simulink model "TrackShift_F1_HEV"  (R2025a)
settings: Solver=FixedStepDiscrete  StartTime=0.0  StopTime=90  FixedStep=0.25  RelTol=1e-3
model workspace (MAT data in the model file):
  TS_BRAKE = [0 0.25 0.5 0.75 1 1.25 1.5 1.75 2 2.25 2.5 2.75 ... (722 elements, 361x2)]
  TS_ENGINE_CAPACITY_L = 1.6
  TS_GAP_S = [0 0.25 0.5 0.75 1 1.25 1.5 1.75 2 2.25 2.5 2.75 ... (722 elements, 361x2)]
  TS_GRADIENT_RAD = [0 0.25 0.5 0.75 1 1.25 1.5 1.75 2 2.25 2.5 2.75 ... (722 elements, 361x2)]
  TS_HANDOVER_SOURCE = 'handover.rar / handover/export/models (production logistic models)'
  TS_SAMPLE_TIME_S = 0.25
  TS_SPEED_KPH = [0 0.25 0.5 0.75 1 1.25 1.5 1.75 2 2.25 2.5 2.75 ... (722 elements, 361x2)]
  TS_THROTTLE = [0 0.25 0.5 0.75 1 1.25 1.5 1.75 2 2.25 2.5 2.75 ... (722 elements, 361x2)]
  TS_TRACK_POS_M = [0 0.25 0.5 0.75 1 1.25 1.5 1.75 2 2.25 2.5 2.75 ... (722 elements, 361x2)]
(part 2 of 2)

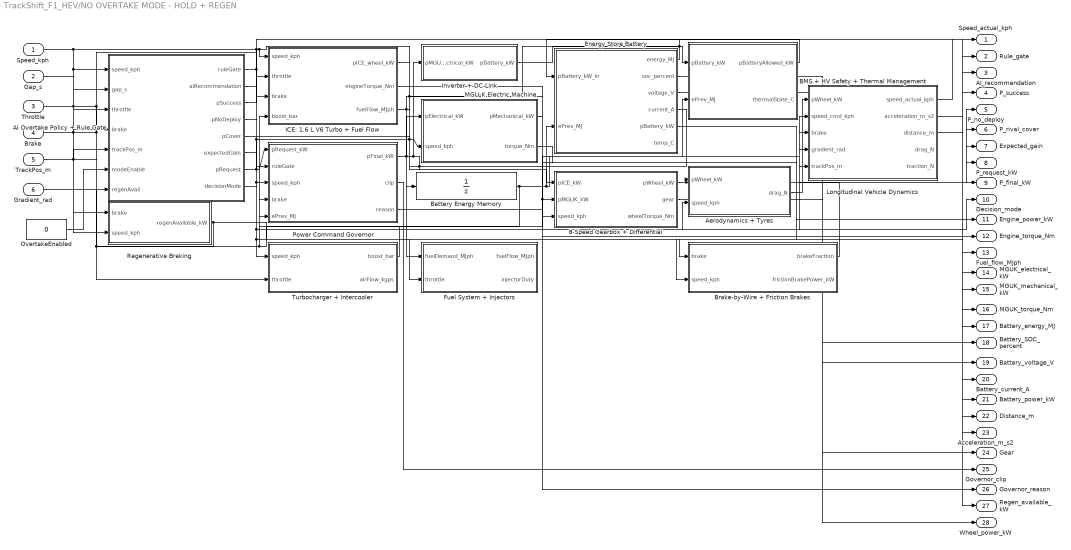
== system TrackShift_F1_HEV/NO OVERTAKE MODE - HOLD + REGEN ==
  Speed_kph : Inport
  Gap_s : Inport  Port=2
  Throttle : Inport  Port=3
  Brake : Inport  Port=4
  TrackPos_m : Inport  Port=5
  Gradient_rad : Inport  Port=6
  8-Speed Gearbox + Differential : MATLAB Function  TreatAsAtomicUnit=on
  AI Overtake Policy + Rule Gate : MATLAB Function  TreatAsAtomicUnit=on
  Aerodynamics + Tyres : MATLAB Function  TreatAsAtomicUnit=on
  BMS + HV Safety + Thermal Management : MATLAB Function  TreatAsAtomicUnit=on
  Battery Energy Memory : UnitDelay  InitialCondition=11.52  SampleTime=0.25  HasFrameUpgradeWarning=on
  Brake-by-Wire + Friction Brakes : MATLAB Function  TreatAsAtomicUnit=on
  Energy Store Battery : MATLAB Function  TreatAsAtomicUnit=on
  Fuel System + Injectors : MATLAB Function  TreatAsAtomicUnit=on
  ICE: 1.6 L V6 Turbo + Fuel Flow : MATLAB Function  TreatAsAtomicUnit=on
  Inverter + DC Link : MATLAB Function  TreatAsAtomicUnit=on
  Longitudinal Vehicle Dynamics : MATLAB Function  TreatAsAtomicUnit=on
  MGU-K Electric Machine : MATLAB Function  TreatAsAtomicUnit=on
  OvertakeEnabled : Constant  Value=0
  Power Command Governor : MATLAB Function  TreatAsAtomicUnit=on
  Regenerative Braking : MATLAB Function  TreatAsAtomicUnit=on
  Turbocharger + Intercooler : MATLAB Function  TreatAsAtomicUnit=on
  Speed_actual_kph : Outport
  Rule_gate : Outport  Port=2
  AI_recommendation : Outport  Port=3
  P_success : Outport  Port=4
  P_no_deploy : Outport  Port=5
  P_rival_cover : Outport  Port=6
  Expected_gain : Outport  Port=7
  P_request_kW : Outport  Port=8
  P_final_kW : Outport  Port=9
  Decision_mode : Outport  Port=10
  Engine_power_kW : Outport  Port=11
  Engine_torque_Nm : Outport  Port=12
  Fuel_flow_MJph : Outport  Port=13
  MGUK_electrical_kW : Outport  Port=14
  MGUK_mechanical_kW : Outport  Port=15
  MGUK_torque_Nm : Outport  Port=16
  Battery_energy_MJ : Outport  Port=17
  Battery_SOC_percent : Outport  Port=18
  Battery_voltage_V : Outport  Port=19
  Battery_current_A : Outport  Port=20
  Battery_power_kW : Outport  Port=21
  Distance_m : Outport  Port=22
  Acceleration_m_s2 : Outport  Port=23
  Gear : Outport  Port=24
  Governor_clip : Outport  Port=25
  Governor_reason : Outport  Port=26
  Regen_available_kW : Outport  Port=27
  Wheel_power_kW : Outport  Port=28
  wires:
  ? -> ?
  Speed_kph/1 -> AI Overtake Policy + Rule Gate/1(speed_kph), Regenerative Braking/2(speed_kph), Turbocharger + Intercooler/1(speed_kph), Brake-by-Wire + Friction Brakes/2(speed_kph), Aerodynamics + Tyres/2(speed_kph), Power Command Governor/3(speed_kph), MGU-K Electric Machine/2(speed_kph), 8-Speed Gearbox + Differential/3(speed_kph), ICE: 1.6 L V6 Turbo + Fuel Flow/1(speed_kph), Longitudinal Vehicle Dynamics/2(speed_cmd_kph)
  Gap_s/1 -> AI Overtake Policy + Rule Gate/2(gap_s)
  Throttle/1 -> Turbocharger + Intercooler/2(throttle), Fuel System + Injectors/2(throttle), ICE: 1.6 L V6 Turbo + Fuel Flow/2(throttle), AI Overtake Policy + Rule Gate/3(throttle)
  Brake/1 -> Power Command Governor/4(brake), Brake-by-Wire + Friction Brakes/1(brake), ICE: 1.6 L V6 Turbo + Fuel Flow/3(brake), AI Overtake Policy + Rule Gate/4(brake), Regenerative Braking/1(brake)
  TrackPos_m/1 -> AI Overtake Policy + Rule Gate/5(trackPos_m), Longitudinal Vehicle Dynamics/5(trackPos_m)
  OvertakeEnabled/1 -> AI Overtake Policy + Rule Gate/6(modeEnable)
  Regenerative Braking/1(regenAvailable_kW) -> AI Overtake Policy + Rule Gate/7(regenAvail), Regen_available_kW/1
  Turbocharger + Intercooler/1(boost_bar) -> ICE: 1.6 L V6 Turbo + Fuel Flow/4(boost_bar)
  ICE: 1.6 L V6 Turbo + Fuel Flow/3(fuelFlow_MJph) -> Fuel System + Injectors/1(fuelDemand_MJph), Fuel_flow_MJph/1
  AI Overtake Policy + Rule Gate/7(pRequest) -> Power Command Governor/1(pRequest_kW), P_request_kW/1
  AI Overtake Policy + Rule Gate/1(ruleGate) -> Power Command Governor/2(ruleGate), Rule_gate/1
  Battery Energy Memory/1 -> Energy Store Battery/2(ePrev_MJ), BMS + HV Safety + Thermal Management/2(ePrev_MJ), Power Command Governor/5(ePrev_MJ)
  Power Command Governor/1(pFinal_kW) -> P_final_kW/1, MGUK_electrical_kW/1, Inverter + DC Link/1(pMGUK_electrical_kW), MGU-K Electric Machine/1(pElectrical_kW)
  Inverter + DC Link/1(pBattery_kW) -> BMS + HV Safety + Thermal Management/1(pBattery_kW)
  BMS + HV Safety + Thermal Management/1(pBatteryAllowed_kW) -> Energy Store Battery/1(pBattery_kW_in)
  Energy Store Battery/1(energy_MJ) -> Battery Energy Memory/1, Battery_energy_MJ/1
  ICE: 1.6 L V6 Turbo + Fuel Flow/1(pICE_wheel_kW) -> 8-Speed Gearbox + Differential/1(pICE_kW), Engine_power_kW/1
  MGU-K Electric Machine/1(pMechanical_kW) -> 8-Speed Gearbox + Differential/2(pMGUK_kW), MGUK_mechanical_kW/1
  8-Speed Gearbox + Differential/1(pWheel_kW) -> Aerodynamics + Tyres/1(pWheel_kW), Wheel_power_kW/1
  Aerodynamics + Tyres/1(drag_N) -> Longitudinal Vehicle Dynamics/1(pWheel_kW)
  Brake-by-Wire + Friction Brakes/1(brakeFraction) -> Longitudinal Vehicle Dynamics/3(brake)
  Gradient_rad/1 -> Longitudinal Vehicle Dynamics/4(gradient_rad)
  Longitudinal Vehicle Dynamics/1(speed_actual_kph) -> Speed_actual_kph/1
  AI Overtake Policy + Rule Gate/2(aiRecommendation) -> AI_recommendation/1
  AI Overtake Policy + Rule Gate/3(pSuccess) -> P_success/1
  AI Overtake Policy + Rule Gate/4(pNoDeploy) -> P_no_deploy/1
  AI Overtake Policy + Rule Gate/5(pCover) -> P_rival_cover/1
  AI Overtake Policy + Rule Gate/6(expectedGain) -> Expected_gain/1
  AI Overtake Policy + Rule Gate/8(decisionMode) -> Decision_mode/1
  ICE: 1.6 L V6 Turbo + Fuel Flow/2(engineTorque_Nm) -> Engine_torque_Nm/1
  MGU-K Electric Machine/2(torque_Nm) -> MGUK_torque_Nm/1
  Energy Store Battery/2(soc_percent) -> Battery_SOC_percent/1
  Energy Store Battery/3(voltage_V) -> Battery_voltage_V/1
  Energy Store Battery/4(current_A) -> Battery_current_A/1
  Energy Store Battery/5(pBattery_kW) -> Battery_power_kW/1
  Longitudinal Vehicle Dynamics/3(distance_m) -> Distance_m/1
  Longitudinal Vehicle Dynamics/2(acceleration_m_s2) -> Acceleration_m_s2/1
  8-Speed Gearbox + Differential/2(gear) -> Gear/1
  Power Command Governor/2(clip) -> Governor_clip/1
  Power Command Governor/3(reason) -> Governor_reason/1

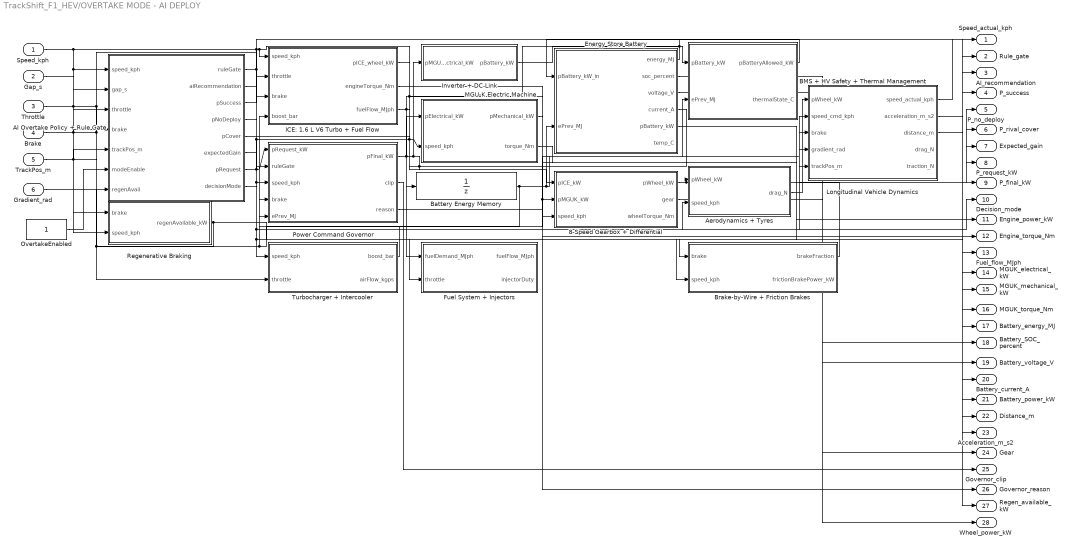
== system TrackShift_F1_HEV/OVERTAKE MODE - AI DEPLOY ==
  Speed_kph : Inport
  Gap_s : Inport  Port=2
  Throttle : Inport  Port=3
  Brake : Inport  Port=4
  TrackPos_m : Inport  Port=5
  Gradient_rad : Inport  Port=6
  8-Speed Gearbox + Differential : MATLAB Function  TreatAsAtomicUnit=on
  AI Overtake Policy + Rule Gate : MATLAB Function  TreatAsAtomicUnit=on
  Aerodynamics + Tyres : MATLAB Function  TreatAsAtomicUnit=on
  BMS + HV Safety + Thermal Management : MATLAB Function  TreatAsAtomicUnit=on
  Battery Energy Memory : UnitDelay  InitialCondition=11.52  SampleTime=0.25  HasFrameUpgradeWarning=on
  Brake-by-Wire + Friction Brakes : MATLAB Function  TreatAsAtomicUnit=on
  Energy Store Battery : MATLAB Function  TreatAsAtomicUnit=on
  Fuel System + Injectors : MATLAB Function  TreatAsAtomicUnit=on
  ICE: 1.6 L V6 Turbo + Fuel Flow : MATLAB Function  TreatAsAtomicUnit=on
  Inverter + DC Link : MATLAB Function  TreatAsAtomicUnit=on
  Longitudinal Vehicle Dynamics : MATLAB Function  TreatAsAtomicUnit=on
  MGU-K Electric Machine : MATLAB Function  TreatAsAtomicUnit=on
  OvertakeEnabled : Constant
  Power Command Governor : MATLAB Function  TreatAsAtomicUnit=on
  Regenerative Braking : MATLAB Function  TreatAsAtomicUnit=on
  Turbocharger + Intercooler : MATLAB Function  TreatAsAtomicUnit=on
  Speed_actual_kph : Outport
  Rule_gate : Outport  Port=2
  AI_recommendation : Outport  Port=3
  P_success : Outport  Port=4
  P_no_deploy : Outport  Port=5
  P_rival_cover : Outport  Port=6
  Expected_gain : Outport  Port=7
  P_request_kW : Outport  Port=8
  P_final_kW : Outport  Port=9
  Decision_mode : Outport  Port=10
  Engine_power_kW : Outport  Port=11
  Engine_torque_Nm : Outport  Port=12
  Fuel_flow_MJph : Outport  Port=13
  MGUK_electrical_kW : Outport  Port=14
  MGUK_mechanical_kW : Outport  Port=15
  MGUK_torque_Nm : Outport  Port=16
  Battery_energy_MJ : Outport  Port=17
  Battery_SOC_percent : Outport  Port=18
  Battery_voltage_V : Outport  Port=19
  Battery_current_A : Outport  Port=20
  Battery_power_kW : Outport  Port=21
  Distance_m : Outport  Port=22
  Acceleration_m_s2 : Outport  Port=23
  Gear : Outport  Port=24
  Governor_clip : Outport  Port=25
  Governor_reason : Outport  Port=26
  Regen_available_kW : Outport  Port=27
  Wheel_power_kW : Outport  Port=28
  wires:
  ? -> ?
  Speed_kph/1 -> AI Overtake Policy + Rule Gate/1(speed_kph), Regenerative Braking/2(speed_kph), Turbocharger + Intercooler/1(speed_kph), Brake-by-Wire + Friction Brakes/2(speed_kph), Aerodynamics + Tyres/2(speed_kph), Power Command Governor/3(speed_kph), MGU-K Electric Machine/2(speed_kph), 8-Speed Gearbox + Differential/3(speed_kph), ICE: 1.6 L V6 Turbo + Fuel Flow/1(speed_kph), Longitudinal Vehicle Dynamics/2(speed_cmd_kph)
  Gap_s/1 -> AI Overtake Policy + Rule Gate/2(gap_s)
  Throttle/1 -> Turbocharger + Intercooler/2(throttle), Fuel System + Injectors/2(throttle), ICE: 1.6 L V6 Turbo + Fuel Flow/2(throttle), AI Overtake Policy + Rule Gate/3(throttle)
  Brake/1 -> Power Command Governor/4(brake), Brake-by-Wire + Friction Brakes/1(brake), ICE: 1.6 L V6 Turbo + Fuel Flow/3(brake), AI Overtake Policy + Rule Gate/4(brake), Regenerative Braking/1(brake)
  TrackPos_m/1 -> AI Overtake Policy + Rule Gate/5(trackPos_m), Longitudinal Vehicle Dynamics/5(trackPos_m)
  OvertakeEnabled/1 -> AI Overtake Policy + Rule Gate/6(modeEnable)
  Regenerative Braking/1(regenAvailable_kW) -> AI Overtake Policy + Rule Gate/7(regenAvail), Regen_available_kW/1
  Turbocharger + Intercooler/1(boost_bar) -> ICE: 1.6 L V6 Turbo + Fuel Flow/4(boost_bar)
  ICE: 1.6 L V6 Turbo + Fuel Flow/3(fuelFlow_MJph) -> Fuel System + Injectors/1(fuelDemand_MJph), Fuel_flow_MJph/1
  AI Overtake Policy + Rule Gate/7(pRequest) -> Power Command Governor/1(pRequest_kW), P_request_kW/1
  AI Overtake Policy + Rule Gate/1(ruleGate) -> Power Command Governor/2(ruleGate), Rule_gate/1
  Battery Energy Memory/1 -> Energy Store Battery/2(ePrev_MJ), BMS + HV Safety + Thermal Management/2(ePrev_MJ), Power Command Governor/5(ePrev_MJ)
  Power Command Governor/1(pFinal_kW) -> P_final_kW/1, MGUK_electrical_kW/1, Inverter + DC Link/1(pMGUK_electrical_kW), MGU-K Electric Machine/1(pElectrical_kW)
  Inverter + DC Link/1(pBattery_kW) -> BMS + HV Safety + Thermal Management/1(pBattery_kW)
  BMS + HV Safety + Thermal Management/1(pBatteryAllowed_kW) -> Energy Store Battery/1(pBattery_kW_in)
  Energy Store Battery/1(energy_MJ) -> Battery Energy Memory/1, Battery_energy_MJ/1
  ICE: 1.6 L V6 Turbo + Fuel Flow/1(pICE_wheel_kW) -> 8-Speed Gearbox + Differential/1(pICE_kW), Engine_power_kW/1
  MGU-K Electric Machine/1(pMechanical_kW) -> 8-Speed Gearbox + Differential/2(pMGUK_kW), MGUK_mechanical_kW/1
  8-Speed Gearbox + Differential/1(pWheel_kW) -> Aerodynamics + Tyres/1(pWheel_kW), Wheel_power_kW/1
  Aerodynamics + Tyres/1(drag_N) -> Longitudinal Vehicle Dynamics/1(pWheel_kW)
  Brake-by-Wire + Friction Brakes/1(brakeFraction) -> Longitudinal Vehicle Dynamics/3(brake)
  Gradient_rad/1 -> Longitudinal Vehicle Dynamics/4(gradient_rad)
  Longitudinal Vehicle Dynamics/1(speed_actual_kph) -> Speed_actual_kph/1
  AI Overtake Policy + Rule Gate/2(aiRecommendation) -> AI_recommendation/1
  AI Overtake Policy + Rule Gate/3(pSuccess) -> P_success/1
  AI Overtake Policy + Rule Gate/4(pNoDeploy) -> P_no_deploy/1
  AI Overtake Policy + Rule Gate/5(pCover) -> P_rival_cover/1
  AI Overtake Policy + Rule Gate/6(expectedGain) -> Expected_gain/1
  AI Overtake Policy + Rule Gate/8(decisionMode) -> Decision_mode/1
  ICE: 1.6 L V6 Turbo + Fuel Flow/2(engineTorque_Nm) -> Engine_torque_Nm/1
  MGU-K Electric Machine/2(torque_Nm) -> MGUK_torque_Nm/1
  Energy Store Battery/2(soc_percent) -> Battery_SOC_percent/1
  Energy Store Battery/3(voltage_V) -> Battery_voltage_V/1
  Energy Store Battery/4(current_A) -> Battery_current_A/1
  Energy Store Battery/5(pBattery_kW) -> Battery_power_kW/1
  Longitudinal Vehicle Dynamics/3(distance_m) -> Distance_m/1
  Longitudinal Vehicle Dynamics/2(acceleration_m_s2) -> Acceleration_m_s2/1
  8-Speed Gearbox + Differential/2(gear) -> Gear/1
  Power Command Governor/2(clip) -> Governor_clip/1
  Power Command Governor/3(reason) -> Governor_reason/1

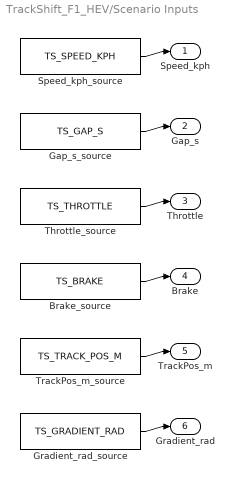
== system TrackShift_F1_HEV/Scenario Inputs ==
  Brake_source : FromWorkspace  VariableName=TS_BRAKE
  Gap_s_source : FromWorkspace  VariableName=TS_GAP_S
  Gradient_rad_source : FromWorkspace  VariableName=TS_GRADIENT_RAD
  Speed_kph_source : FromWorkspace  VariableName=TS_SPEED_KPH
  Throttle_source : FromWorkspace  VariableName=TS_THROTTLE
  TrackPos_m_source : FromWorkspace  VariableName=TS_TRACK_POS_M
  Speed_kph : Outport
  Gap_s : Outport  Port=2
  Throttle : Outport  Port=3
  Brake : Outport  Port=4
  TrackPos_m : Outport  Port=5
  Gradient_rad : Outport  Port=6
  wires:
  ? -> ?
  Speed_kph_source/1 -> Speed_kph/1
  Gap_s_source/1 -> Gap_s/1
  Throttle_source/1 -> Throttle/1
  Brake_source/1 -> Brake/1
  TrackPos_m_source/1 -> TrackPos_m/1
  Gradient_rad_source/1 -> Gradient_rad/1

== matlab function TrackShift_F1_HEV/OVERTAKE MODE - AI DEPLOY/Energy Store Battery ==
  data: pBattery_kW_in input; energy_MJ output; ePrev_MJ input; soc_percent output; voltage_V output; current_A output; pBattery_kW output; temp_C output
function [energy_MJ,soc_percent,voltage_V,current_A,pBattery_kW,temp_C] = f(pBattery_kW_in,ePrev_MJ)
capacity = 14.4; eMin = capacity*0.20; eMax = capacity*0.95; dt = 0.25;
e = min(max(ePrev_MJ-pBattery_kW_in*dt/1000,eMin),eMax); soc = min(max(e/capacity,0),1);
voc = 400*(0.95+0.10*soc); r = 0.08; pW = pBattery_kW_in*1000;
disc = max(voc^2-4*r*pW,0); current_A = (voc-sqrt(disc))/(2*r); voltage_V = max(50,voc-r*current_A);
current_A = pW/voltage_V; temp_C = 35+0.001*abs(pBattery_kW_in);
energy_MJ = e; soc_percent = 100*soc; pBattery_kW = pBattery_kW_in;
end

== matlab function TrackShift_F1_HEV/OVERTAKE MODE - AI DEPLOY/BMS + HV Safety + Thermal Management ==
  data: pBattery_kW input; pBatteryAllowed_kW output; ePrev_MJ input; thermalState_C output
function [pBatteryAllowed_kW,thermalState_C] = f(pBattery_kW,ePrev_MJ)
% Battery-management, HV interlock and thermal protection layer.
capacity_MJ = 14.4; eMin_MJ = 0.20*capacity_MJ; eMax_MJ = 0.95*capacity_MJ;
if ePrev_MJ <= eMin_MJ && pBattery_kW > 0, pBatteryAllowed_kW = 0;
elseif ePrev_MJ >= eMax_MJ && pBattery_kW < 0, pBatteryAllowed_kW = 0;
else, pBatteryAllowed_kW = min(max(pBattery_kW,-180),350); end
thermalState_C = 35+0.001*abs(pBatteryAllowed_kW);
end

== matlab function TrackShift_F1_HEV/OVERTAKE MODE - AI DEPLOY/8-Speed Gearbox + Differential ==
  data: pICE_kW input; pWheel_kW output; pMGUK_kW input; speed_kph input; gear output; wheelTorque_Nm output
function [pWheel_kW,gear,wheelTorque_Nm] = f(pICE_kW,pMGUK_kW,speed_kph)
gear = 1+floor(min(max((speed_kph-70)/34,0),7));
pWheel_kW = (pICE_kW+pMGUK_kW)*0.95;
wheelTorque_Nm = pWheel_kW*1000/max(speed_kph/3.6,1);
end

== matlab function TrackShift_F1_HEV/OVERTAKE MODE - AI DEPLOY/Aerodynamics + Tyres ==
  data: pWheel_kW input; drag_N output; speed_kph input
function drag_N = f(pWheel_kW,speed_kph)
% Aerodynamic drag feedback is reported as a component signal.
rho = 1.225; cda = 0.925; v = max(speed_kph/3.6,1);
drag_N = 0.5*rho*cda*v^2;
end

== matlab function TrackShift_F1_HEV/OVERTAKE MODE - AI DEPLOY/Brake-by-Wire + Friction Brakes ==
  data: brake input; brakeFraction output; speed_kph input; frictionBrakePower_kW output
function [brakeFraction,frictionBrakePower_kW] = f(brake,speed_kph)
% Brake-by-wire allocation leaves regenerative braking on the parallel path.
brakeFraction = min(max(brake,0),1);
frictionBrakePower_kW = brakeFraction*max(speed_kph,0)*18.0;
end

== matlab function TrackShift_F1_HEV/OVERTAKE MODE - AI DEPLOY/Longitudinal Vehicle Dynamics ==
  data: pWheel_kW input; speed_actual_kph output; speed_cmd_kph input; brake input; gradient_rad input; trackPos_m input; acceleration_m_s2 output; distance_m output; drag_N output; traction_N output
function [speed_actual_kph,acceleration_m_s2,distance_m,drag_N,traction_N] = f(pWheel_kW,speed_cmd_kph,brake,gradient_rad,trackPos_m)
mass = 803; g = 9.81; rho = 1.225; cda = 0.925; v = max(speed_cmd_kph/3.6,1);
traction_N = pWheel_kW*1000/v; drag_N = 0.5*rho*cda*v^2;
roll_N = 0.30*mass; grade_N = mass*g*sin(gradient_rad); brake_N = min(max(brake,0),1)*18000;
acceleration_m_s2 = min(max((traction_N-drag_N-roll_N-grade_N-brake_N)/mass,-12),12);
speed_actual_kph = max(0,speed_cmd_kph+3.6*0.25*acceleration_m_s2);
distance_m = trackPos_m+speed_actual_kph/3.6*0.25;
end

== matlab function TrackShift_F1_HEV/NO OVERTAKE MODE - HOLD + REGEN/AI Overtake Policy + Rule Gate ==
  data: speed_kph input; ruleGate output; gap_s input; throttle input; brake input; trackPos_m input; modeEnable input; regenAvail input; aiRecommendation output; pSuccess output; pNoDeploy output; pCover output; expectedGain output; pRequest output; decisionMode output
function [ruleGate,aiRecommendation,pSuccess,pNoDeploy,pCover,expectedGain,pRequest,decisionMode] = f(speed_kph,gap_s,throttle,brake,trackPos_m,modeEnable,regenAvail)
% Production coefficients embedded from handover.rar.
zone = [-0.7075777832923592;-6.026485573777835;-0.04895038433595806;-0.13455035383372793;-0.11816067407748346;1.055251955308986;1.5560826217886794;0.1588318525718114;0.4247931092675822;0.21790016690200298];
cover = [-1.940559726452234;-0.27364141130466757;0.6096490191848467;0.05772237959270659;-0.00991799169367214;-0.2114018519558647;-0.01166365647510053;4.432492080111768;1.679664114999441;-0.3868757212959778;-0.4455625799447156];
lap = [-0.8405861024010692;-1.9463537472006074;-0.08489712734227542];
lapLength = 5000.0; zoneLen = 0.45; nextZone = 1.5; isLast = 0.0; tyreDelta = 0.0;
lapPhase = min(max(trackPos_m/lapLength,0),1);
p00 = logistic(zone,[1;gap_s;tyreDelta;0;0;0;zoneLen;nextZone;isLast;0]);
p10 = logistic(zone,[1;gap_s;tyreDelta;1;0;1;zoneLen;nextZone;isLast;gap_s]);
p01 = logistic(zone,[1;gap_s;tyreDelta;0;1;0;zoneLen;nextZone;isLast;0]);
p11 = logistic(zone,[1;gap_s;tyreDelta;1;1;0;zoneLen;nextZone;isLast;gap_s]);
pCover = logistic(cover,[1;2.5;0;0.5;5;gap_s;tyreDelta;zoneLen;isLast;lapPhase;0]);
pSuccess = (1-pCover)*p10+pCover*p11;
pNoDeploy = (1-pCover)*p00+pCover*p01;
gainUnmatched = p10-p00; gainMatched = p11-p01;
expectedGain = (1-pCover)*gainUnmatched+pCover*gainMatched;
aiRecommendation = modeEnable > 0 && expectedGain >= 0.04;
ruleGate = modeEnable > 0 && gap_s <= 0.90 && trackPos_m >= 1150 && trackPos_m <= 1650;
if ruleGate && aiRecommendation && speed_kph > 215
    decisionMode = 1; pRequest = 275;
elseif brake >= 0.22 && regenAvail > 0
    decisionMode = -1; pRequest = -120;
else
    decisionMode = 0; pRequest = 0;
end
end
function p = logistic(b,x)
p = min(max(1/(1+exp(-(b'*x))),0),1);
end

== matlab function TrackShift_F1_HEV/NO OVERTAKE MODE - HOLD + REGEN/Regenerative Braking ==
  data: brake input; regenAvailable_kW output; speed_kph input
function regenAvailable_kW = f(brake,speed_kph)
% Rear-axle regenerative braking availability, capped for this reference model.
regenAvailable_kW = min(max(brake,0)*max(speed_kph,0)*0.40,180);
end

== matlab function TrackShift_F1_HEV/OVERTAKE MODE - AI DEPLOY/Regenerative Braking ==
  data: brake input; regenAvailable_kW output; speed_kph input
function regenAvailable_kW = f(brake,speed_kph)
% Rear-axle regenerative braking availability, capped for this reference model.
regenAvailable_kW = min(max(brake,0)*max(speed_kph,0)*0.40,180);
end

== matlab function TrackShift_F1_HEV/NO OVERTAKE MODE - HOLD + REGEN/ICE: 1.6 L V6 Turbo + Fuel Flow ==
  data: speed_kph input; pICE_wheel_kW output; throttle input; brake input; boost_bar input; engineTorque_Nm output; fuelFlow_MJph output
function [pICE_wheel_kW,engineTorque_Nm,fuelFlow_MJph] = f(speed_kph,throttle,brake,boost_bar)
rpm = min(max(speed_kph/3.6/0.330*3.20*3.50*60/(2*pi),4000),10500);
baseTorque = min(max(700 + 0.01*(rpm-4000),0),720);
effectiveThrottle = min(max(throttle*(1-brake),0),1);
boostFactor = min(max(0.90+0.025*boost_bar,0.90),1.05);
fuelFlow_MJph = min(3000,165+0.27*rpm);
pFuel_kW = fuelFlow_MJph*1000/3600;
omega = rpm*2*pi/60;
pShaft_kW = min(pFuel_kW*0.55*effectiveThrottle*boostFactor,baseTorque*effectiveThrottle*omega/1000*boostFactor);
engineTorque_Nm = max(0,pShaft_kW*1000/max(omega,1));
pICE_wheel_kW = max(0,pShaft_kW*0.95);
end

== matlab function TrackShift_F1_HEV/NO OVERTAKE MODE - HOLD + REGEN/Turbocharger + Intercooler ==
  data: speed_kph input; boost_bar output; throttle input; airFlow_kgps output
function [boost_bar,airFlow_kgps] = f(speed_kph,throttle)
% Turbocharger compressor/turbine and intercooler signal-level model.
boost_bar = min(max(1.0+0.010*max(speed_kph,0)+2.0*max(throttle,0),1.0),5.0);
airFlow_kgps = min(max(0.002*max(speed_kph,0)*max(throttle,0),0),1.6);
end

== matlab function TrackShift_F1_HEV/NO OVERTAKE MODE - HOLD + REGEN/Fuel System + Injectors ==
  data: fuelDemand_MJph input; fuelFlow_MJph output; throttle input; injectorDuty output
function [fuelFlow_MJph,injectorDuty] = f(fuelDemand_MJph,throttle)
% Fuel rail, injectors and sustainable-fuel delivery monitor.
fuelFlow_MJph = max(fuelDemand_MJph,0);
injectorDuty = min(max(throttle,0),1);
end

== matlab function TrackShift_F1_HEV/NO OVERTAKE MODE - HOLD + REGEN/Power Command Governor ==
  data: pRequest_kW input; pFinal_kW output; ruleGate input; speed_kph input; brake input; ePrev_MJ input; clip output; reason output
function [pFinal_kW,clip,reason] = f(pRequest_kW,ruleGate,speed_kph,brake,ePrev_MJ)
cap = 350; dt = 0.25; eMin = 2.88; swing = 4.0;
omega = max(1,speed_kph/3.6/0.330*3.50); physical = min(cap,500*omega/1000);
if pRequest_kW > 0 && ruleGate > 0
    if speed_kph < 340, reg = 350; elseif speed_kph < 345, reg = 100*(345-speed_kph)/5; else, reg = 0; end
    energyLimit = max(0,(ePrev_MJ-max(eMin,ePrev_MJ-swing)))*1000/dt*0.97*0.96;
    pFinal_kW = min([pRequest_kW,reg,physical,350,energyLimit]); reason = 0;
elseif pRequest_kW < 0 && brake >= 0.22
    pFinal_kW = -min(abs(pRequest_kW),180); reason = 2;
else
    pFinal_kW = 0; reason = 1;
end
clip = double(abs(pFinal_kW-pRequest_kW)>1e-9);
end

== matlab function TrackShift_F1_HEV/NO OVERTAKE MODE - HOLD + REGEN/Inverter + DC Link ==
  data: pMGUK_electrical_kW input; pBattery_kW output
function pBattery_kW = f(pMGUK_electrical_kW)
if pMGUK_electrical_kW >= 0, pBattery_kW = pMGUK_electrical_kW/0.97; else, pBattery_kW = pMGUK_electrical_kW*0.97; end
end

== matlab function TrackShift_F1_HEV/NO OVERTAKE MODE - HOLD + REGEN/MGU-K Electric Machine ==
  data: pElectrical_kW input; pMechanical_kW output; speed_kph input; torque_Nm output
function [pMechanical_kW,torque_Nm] = f(pElectrical_kW,speed_kph)
omega = max(1,speed_kph/3.6/0.330*3.50); eta = 0.96;
if pElectrical_kW >= 0, pMechanical_kW = pElectrical_kW*eta; else, pMechanical_kW = pElectrical_kW/max(eta,1e-6); end
torque_Nm = min(max(pMechanical_kW*1000/omega,-500),500);
pMechanical_kW = torque_Nm*omega/1000;
end

== matlab function TrackShift_F1_HEV/NO OVERTAKE MODE - HOLD + REGEN/Energy Store Battery ==
  data: pBattery_kW_in input; energy_MJ output; ePrev_MJ input; soc_percent output; voltage_V output; current_A output; pBattery_kW output; temp_C output
function [energy_MJ,soc_percent,voltage_V,current_A,pBattery_kW,temp_C] = f(pBattery_kW_in,ePrev_MJ)
capacity = 14.4; eMin = capacity*0.20; eMax = capacity*0.95; dt = 0.25;
e = min(max(ePrev_MJ-pBattery_kW_in*dt/1000,eMin),eMax); soc = min(max(e/capacity,0),1);
voc = 400*(0.95+0.10*soc); r = 0.08; pW = pBattery_kW_in*1000;
disc = max(voc^2-4*r*pW,0); current_A = (voc-sqrt(disc))/(2*r); voltage_V = max(50,voc-r*current_A);
current_A = pW/voltage_V; temp_C = 35+0.001*abs(pBattery_kW_in);
energy_MJ = e; soc_percent = 100*soc; pBattery_kW = pBattery_kW_in;
end

== matlab function TrackShift_F1_HEV/NO OVERTAKE MODE - HOLD + REGEN/BMS + HV Safety + Thermal Management ==
  data: pBattery_kW input; pBatteryAllowed_kW output; ePrev_MJ input; thermalState_C output
function [pBatteryAllowed_kW,thermalState_C] = f(pBattery_kW,ePrev_MJ)
% Battery-management, HV interlock and thermal protection layer.
capacity_MJ = 14.4; eMin_MJ = 0.20*capacity_MJ; eMax_MJ = 0.95*capacity_MJ;
if ePrev_MJ <= eMin_MJ && pBattery_kW > 0, pBatteryAllowed_kW = 0;
elseif ePrev_MJ >= eMax_MJ && pBattery_kW < 0, pBatteryAllowed_kW = 0;
else, pBatteryAllowed_kW = min(max(pBattery_kW,-180),350); end
thermalState_C = 35+0.001*abs(pBatteryAllowed_kW);
end

== matlab function TrackShift_F1_HEV/OVERTAKE MODE - AI DEPLOY/AI Overtake Policy + Rule Gate ==
  data: speed_kph input; ruleGate output; gap_s input; throttle input; brake input; trackPos_m input; modeEnable input; regenAvail input; aiRecommendation output; pSuccess output; pNoDeploy output; pCover output; expectedGain output; pRequest output; decisionMode output
function [ruleGate,aiRecommendation,pSuccess,pNoDeploy,pCover,expectedGain,pRequest,decisionMode] = f(speed_kph,gap_s,throttle,brake,trackPos_m,modeEnable,regenAvail)
% Production coefficients embedded from handover.rar.
zone = [-0.7075777832923592;-6.026485573777835;-0.04895038433595806;-0.13455035383372793;-0.11816067407748346;1.055251955308986;1.5560826217886794;0.1588318525718114;0.4247931092675822;0.21790016690200298];
cover = [-1.940559726452234;-0.27364141130466757;0.6096490191848467;0.05772237959270659;-0.00991799169367214;-0.2114018519558647;-0.01166365647510053;4.432492080111768;1.679664114999441;-0.3868757212959778;-0.4455625799447156];
lap = [-0.8405861024010692;-1.9463537472006074;-0.08489712734227542];
lapLength = 5000.0; zoneLen = 0.45; nextZone = 1.5; isLast = 0.0; tyreDelta = 0.0;
lapPhase = min(max(trackPos_m/lapLength,0),1);
p00 = logistic(zone,[1;gap_s;tyreDelta;0;0;0;zoneLen;nextZone;isLast;0]);
p10 = logistic(zone,[1;gap_s;tyreDelta;1;0;1;zoneLen;nextZone;isLast;gap_s]);
p01 = logistic(zone,[1;gap_s;tyreDelta;0;1;0;zoneLen;nextZone;isLast;0]);
p11 = logistic(zone,[1;gap_s;tyreDelta;1;1;0;zoneLen;nextZone;isLast;gap_s]);
pCover = logistic(cover,[1;2.5;0;0.5;5;gap_s;tyreDelta;zoneLen;isLast;lapPhase;0]);
pSuccess = (1-pCover)*p10+pCover*p11;
pNoDeploy = (1-pCover)*p00+pCover*p01;
gainUnmatched = p10-p00; gainMatched = p11-p01;
expectedGain = (1-pCover)*gainUnmatched+pCover*gainMatched;
aiRecommendation = modeEnable > 0 && expectedGain >= 0.04;
ruleGate = modeEnable > 0 && gap_s <= 0.90 && trackPos_m >= 1150 && trackPos_m <= 1650;
if ruleGate && aiRecommendation && speed_kph > 215
    decisionMode = 1; pRequest = 275;
elseif brake >= 0.22 && regenAvail > 0
    decisionMode = -1; pRequest = -120;
else
    decisionMode = 0; pRequest = 0;
end
end
function p = logistic(b,x)
p = min(max(1/(1+exp(-(b'*x))),0),1);
end

== matlab function TrackShift_F1_HEV/NO OVERTAKE MODE - HOLD + REGEN/8-Speed Gearbox + Differential ==
  data: pICE_kW input; pWheel_kW output; pMGUK_kW input; speed_kph input; gear output; wheelTorque_Nm output
function [pWheel_kW,gear,wheelTorque_Nm] = f(pICE_kW,pMGUK_kW,speed_kph)
gear = 1+floor(min(max((speed_kph-70)/34,0),7));
pWheel_kW = (pICE_kW+pMGUK_kW)*0.95;
wheelTorque_Nm = pWheel_kW*1000/max(speed_kph/3.6,1);
end

== matlab function TrackShift_F1_HEV/NO OVERTAKE MODE - HOLD + REGEN/Aerodynamics + Tyres ==
  data: pWheel_kW input; drag_N output; speed_kph input
function drag_N = f(pWheel_kW,speed_kph)
% Aerodynamic drag feedback is reported as a component signal.
rho = 1.225; cda = 0.925; v = max(speed_kph/3.6,1);
drag_N = 0.5*rho*cda*v^2;
end

== matlab function TrackShift_F1_HEV/NO OVERTAKE MODE - HOLD + REGEN/Brake-by-Wire + Friction Brakes ==
  data: brake input; brakeFraction output; speed_kph input; frictionBrakePower_kW output
function [brakeFraction,frictionBrakePower_kW] = f(brake,speed_kph)
% Brake-by-wire allocation leaves regenerative braking on the parallel path.
brakeFraction = min(max(brake,0),1);
frictionBrakePower_kW = brakeFraction*max(speed_kph,0)*18.0;
end

== matlab function TrackShift_F1_HEV/NO OVERTAKE MODE - HOLD + REGEN/Longitudinal Vehicle Dynamics ==
  data: pWheel_kW input; speed_actual_kph output; speed_cmd_kph input; brake input; gradient_rad input; trackPos_m input; acceleration_m_s2 output; distance_m output; drag_N output; traction_N output
function [speed_actual_kph,acceleration_m_s2,distance_m,drag_N,traction_N] = f(pWheel_kW,speed_cmd_kph,brake,gradient_rad,trackPos_m)
mass = 803; g = 9.81; rho = 1.225; cda = 0.925; v = max(speed_cmd_kph/3.6,1);
traction_N = pWheel_kW*1000/v; drag_N = 0.5*rho*cda*v^2;
roll_N = 0.30*mass; grade_N = mass*g*sin(gradient_rad); brake_N = min(max(brake,0),1)*18000;
acceleration_m_s2 = min(max((traction_N-drag_N-roll_N-grade_N-brake_N)/mass,-12),12);
speed_actual_kph = max(0,speed_cmd_kph+3.6*0.25*acceleration_m_s2);
distance_m = trackPos_m+speed_actual_kph/3.6*0.25;
end

== matlab function TrackShift_F1_HEV/OVERTAKE MODE - AI DEPLOY/ICE: 1.6 L V6 Turbo + Fuel Flow ==
  data: speed_kph input; pICE_wheel_kW output; throttle input; brake input; boost_bar input; engineTorque_Nm output; fuelFlow_MJph output
function [pICE_wheel_kW,engineTorque_Nm,fuelFlow_MJph] = f(speed_kph,throttle,brake,boost_bar)
rpm = min(max(speed_kph/3.6/0.330*3.20*3.50*60/(2*pi),4000),10500);
baseTorque = min(max(700 + 0.01*(rpm-4000),0),720);
effectiveThrottle = min(max(throttle*(1-brake),0),1);
boostFactor = min(max(0.90+0.025*boost_bar,0.90),1.05);
fuelFlow_MJph = min(3000,165+0.27*rpm);
pFuel_kW = fuelFlow_MJph*1000/3600;
omega = rpm*2*pi/60;
pShaft_kW = min(pFuel_kW*0.55*effectiveThrottle*boostFactor,baseTorque*effectiveThrottle*omega/1000*boostFactor);
engineTorque_Nm = max(0,pShaft_kW*1000/max(omega,1));
pICE_wheel_kW = max(0,pShaft_kW*0.95);
end

== matlab function TrackShift_F1_HEV/OVERTAKE MODE - AI DEPLOY/Turbocharger + Intercooler ==
  data: speed_kph input; boost_bar output; throttle input; airFlow_kgps output
function [boost_bar,airFlow_kgps] = f(speed_kph,throttle)
% Turbocharger compressor/turbine and intercooler signal-level model.
boost_bar = min(max(1.0+0.010*max(speed_kph,0)+2.0*max(throttle,0),1.0),5.0);
airFlow_kgps = min(max(0.002*max(speed_kph,0)*max(throttle,0),0),1.6);
end

== matlab function TrackShift_F1_HEV/OVERTAKE MODE - AI DEPLOY/Fuel System + Injectors ==
  data: fuelDemand_MJph input; fuelFlow_MJph output; throttle input; injectorDuty output
function [fuelFlow_MJph,injectorDuty] = f(fuelDemand_MJph,throttle)
% Fuel rail, injectors and sustainable-fuel delivery monitor.
fuelFlow_MJph = max(fuelDemand_MJph,0);
injectorDuty = min(max(throttle,0),1);
end

== matlab function TrackShift_F1_HEV/OVERTAKE MODE - AI DEPLOY/Power Command Governor ==
  data: pRequest_kW input; pFinal_kW output; ruleGate input; speed_kph input; brake input; ePrev_MJ input; clip output; reason output
function [pFinal_kW,clip,reason] = f(pRequest_kW,ruleGate,speed_kph,brake,ePrev_MJ)
cap = 350; dt = 0.25; eMin = 2.88; swing = 4.0;
omega = max(1,speed_kph/3.6/0.330*3.50); physical = min(cap,500*omega/1000);
if pRequest_kW > 0 && ruleGate > 0
    if speed_kph < 340, reg = 350; elseif speed_kph < 345, reg = 100*(345-speed_kph)/5; else, reg = 0; end
    energyLimit = max(0,(ePrev_MJ-max(eMin,ePrev_MJ-swing)))*1000/dt*0.97*0.96;
    pFinal_kW = min([pRequest_kW,reg,physical,350,energyLimit]); reason = 0;
elseif pRequest_kW < 0 && brake >= 0.22
    pFinal_kW = -min(abs(pRequest_kW),180); reason = 2;
else
    pFinal_kW = 0; reason = 1;
end
clip = double(abs(pFinal_kW-pRequest_kW)>1e-9);
end

== matlab function TrackShift_F1_HEV/OVERTAKE MODE - AI DEPLOY/Inverter + DC Link ==
  data: pMGUK_electrical_kW input; pBattery_kW output
function pBattery_kW = f(pMGUK_electrical_kW)
if pMGUK_electrical_kW >= 0, pBattery_kW = pMGUK_electrical_kW/0.97; else, pBattery_kW = pMGUK_electrical_kW*0.97; end
end

== matlab function TrackShift_F1_HEV/OVERTAKE MODE - AI DEPLOY/MGU-K Electric Machine ==
  data: pElectrical_kW input; pMechanical_kW output; speed_kph input; torque_Nm output
function [pMechanical_kW,torque_Nm] = f(pElectrical_kW,speed_kph)
omega = max(1,speed_kph/3.6/0.330*3.50); eta = 0.96;
if pElectrical_kW >= 0, pMechanical_kW = pElectrical_kW*eta; else, pMechanical_kW = pElectrical_kW/max(eta,1e-6); end
torque_Nm = min(max(pMechanical_kW*1000/omega,-500),500);
pMechanical_kW = torque_Nm*omega/1000;
end
